simulink model "SMA_Model"  (R2021b)
settings: Solver=VariableStepAuto  StartTime=0.0  StopTime=50.0  FixedStep=1e-6  RelTol=1e-3
values from neighbouring files (symbols this model uses):
  c_heat = 837.36    [Model_Parameters.m]
  do = 5e-4    (= 0.0005)    [Model_Parameters.m]
  h = 70    [Model_Parameters.m]
  i = 0.8    [Model_Parameters.m]
  Initial_Rm = 1    [Model_Parameters.m]
  Initial_temperature = 100    [Model_Parameters.m]
  Lo = 0.98    [Model_Parameters.m]
  mu_minus = 57    [Model_Parameters.m]
  mu_plus = 72    [Model_Parameters.m]
  ni_minus = 1    [Model_Parameters.m]
  ni_plus = 1    [Model_Parameters.m]
  R = 4.3    [Model_Parameters.m]
  rho = 6450    [Model_Parameters.m]
  sigma_minus = 6    [Model_Parameters.m]
  sigma_plus = 6    [Model_Parameters.m]
  Slider_Friction = 0.11    [Model_Parameters.m]
  T_amb = 20    [Model_Parameters.m]
  v = 24    [Model_Parameters.m]
libraries: fl_lib x7, nesl_utility x3
settings Model: Creator=barag  LastModifiedBy=barag

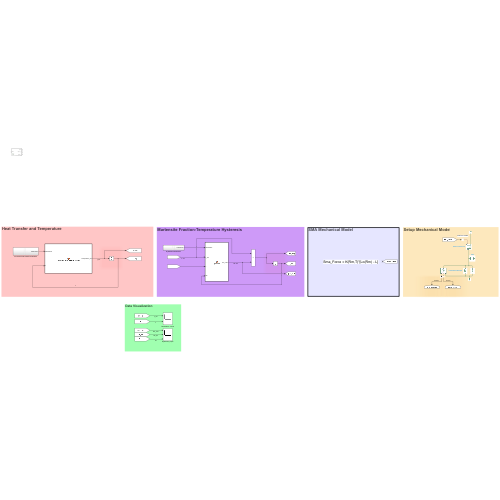
[thumbnail: Simulink's stored preview of the top-level diagram]
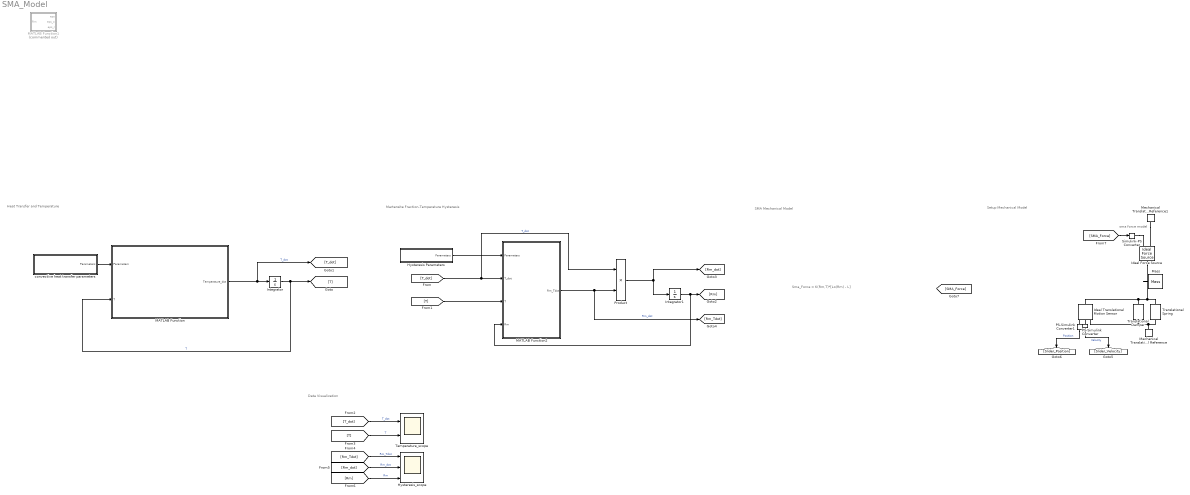
== system SMA_Model ==
  note: Sma_Force = K(Rm,T)*[Lo(Rm) - L]
  note: SMA Mechanical Model
  note: Setup Mechanical Model
  note: sma force model
  note: Data Visualization
  note: Martensite Fraction-Temperature Hysteresis
  note: Heat Transfer and Temperature
  Hysteresis Parameters : Subsystem
  Hysteresis_scope : Scope  NumInputPorts=3
  Ideal Force Source : fl_lib/Mechanical/Mechanical Sources/Ideal Force Source
  Ideal Translational Motion Sensor : fl_lib/Mechanical/Mechanical Sensors/Ideal Translational Motion Sensor  offset=0 m
  Integrator : Integrator  InitialCondition=Initial_temperature
  Integrator1 : Integrator  InitialCondition=Initial_Rm
  MATLAB Function : MATLAB Function  TreatAsAtomicUnit=on
  MATLAB Function1 : MATLAB Function  Commented=on  TreatAsAtomicUnit=on
  MATLAB Function2 : MATLAB Function  TreatAsAtomicUnit=on
  Mass : fl_lib/Mechanical/Translational Elements/Mass  mass=Slider_Mass kg  num_ports=foundation.enum.numPorts2.one  v_specify=off  v_priority=High  v=0 m/s  v_nominal_specify=off  v_nominal_unit=m/s  v_nominal_value=1  f_specify=off  f_priority=None  f=0 N  f_nominal_specify=off  f_nominal_unit=N  f_nominal_value=1
  Mechanical Translational Reference : fl_lib/Mechanical/Translational Elements/Mechanical Translational Reference
  Mechanical Translational Reference1 : fl_lib/Mechanical/Translational Elements/Mechanical Translational Reference
  PS-Simulink Converter : nesl_utility/PS-Simulink Converter  PhysicalDomain=network_engine_domain  SubClassName=ps_output  LeftPortType=input  RightPortType=output  PseudoPeriodic=off  Frequencies=[]  Unit=inherit  AffineConversion=off
      settings: SourceProductBaseCode=PW,SS
  PS-Simulink Converter1 : nesl_utility/PS-Simulink Converter  PhysicalDomain=network_engine_domain  SubClassName=ps_output  LeftPortType=input  RightPortType=output  PseudoPeriodic=off  Frequencies=[]  Unit=inherit  AffineConversion=off
      settings: SourceProductBaseCode=PW,SS
  Product : Product
  Simulink-PS Converter : nesl_utility/Simulink-PS Converter  PhysicalDomain=network_engine_domain  SubClassName=ps_input  LeftPortType=input  RightPortType=output  PseudoPeriodic=off  Frequencies=[]  NoiseDistribution=none  NoiseParameters=[]  Unit=1  AffineConversion=off  FilteringAndDerivatives=provide  SimscapeFilterOrder=1  InputFilterTimeConstant=0.001  UdotUserProvided=0
      settings: SourceProductBaseCode=PW,SS
  Temperature_scope : Scope  NumInputPorts=2
  Translational Damper : fl_lib/Mechanical/Translational Elements/Translational Damper  D=Slider_Friction N/(m/s)  v_specify=off  v_priority=None  v=0 m/s  v_nominal_specify=off  v_nominal_unit=m/s  v_nominal_value=1  f_specify=off  f_priority=None  f=0 N  f_nominal_specify=off  f_nominal_unit=N  f_nominal_value=1
  Translational Spring : fl_lib/Mechanical/Translational Elements/Translational Spring  spr_rate=Spring_Stiff N/m  v_specify=off  v_priority=None  v=0 m/s  v_nominal_specify=off  v_nominal_unit=m/s  v_nominal_value=1  f_specify=off  f_priority=High  f=9 N  f_nominal_specify=off  f_nominal_unit=N  f_nominal_value=1  x_specify=off  x_priority=High  x=0 m  x_nominal_specify=off  x_nominal_unit=m  x_nominal_value=1
  convective heat transfer parameters : Subsystem
  wires:
  MATLAB Function/1(Temperature_dot) -> [T_dot], Integrator/1  "T_dot"
  Integrator/1 -> [T], MATLAB Function/2(T)  "T"
  convective heat transfer parameters/1(Parameters) -> MATLAB Function/1(Parameters)
  Hysteresis Parameters/1(Parameters) -> MATLAB Function2/1(Parameters)
  [T_dot] -> Product/1, MATLAB Function2/2(T_dot)  "T_dot"
  MATLAB Function2/1(Rm_Tdot) -> [Rm_Tdot], Product/2  "Rm_dot"
  [T_dot] -> Temperature_scope/1  "T_dot"
  [T] -> Temperature_scope/2  "T"
  [Rm_Tdot] -> Hysteresis_scope/1  "Rm_Tdot"
  [Rm_dot] -> Hysteresis_scope/2  "Rm_dot"
  [Rm] -> Hysteresis_scope/3  "Rm"
  Integrator1/1 -> [Rm], MATLAB Function2/4(Rm)
  [T] -> MATLAB Function2/3(T)
  Product/1 -> [Rm_dot], Integrator1/1
  PS-Simulink Converter/1 -> [Slider_Velocity]  "Velocity"
  PS-Simulink Converter1/1 -> [Slider_Position]  "Position"
  [SMA_Force] -> Simulink-PS Converter/1
  connections:
  Translational Damper/RConn1 -- Ideal Translational Motion Sensor/RConn1 -- Translational Spring/RConn1 -- Mechanical Translational Reference/LConn1
  Translational Damper/LConn1 -- Ideal Translational Motion Sensor/LConn1 -- Mass/LConn1 -- Ideal Force Source/LConn1 -- Translational Spring/LConn1
  Mechanical Translational Reference1/LConn1 -- Ideal Force Source/RConn2
  PS-Simulink Converter/LConn1 -- Ideal Translational Motion Sensor/RConn2
  PS-Simulink Converter1/LConn1 -- Ideal Translational Motion Sensor/RConn3
  Simulink-PS Converter/RConn1 -- Ideal Force Source/RConn1

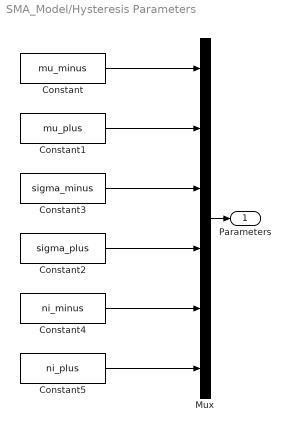
== system SMA_Model/Hysteresis Parameters ==
  Constant : Constant  Value=mu_minus
  Constant1 : Constant  Value=mu_plus
  Constant2 : Constant  Value=sigma_plus
  Constant3 : Constant  Value=sigma_minus
  Constant4 : Constant  Value=ni_minus
  Constant5 : Constant  Value=ni_plus
  Mux : Mux  Inputs=6
  Parameters : Outport
  wires:
  Mux/1 -> Parameters/1
  Constant2/1 -> Mux/4
  Constant/1 -> Mux/1
  Constant4/1 -> Mux/5
  Constant1/1 -> Mux/2
  Constant5/1 -> Mux/6
  Constant3/1 -> Mux/3

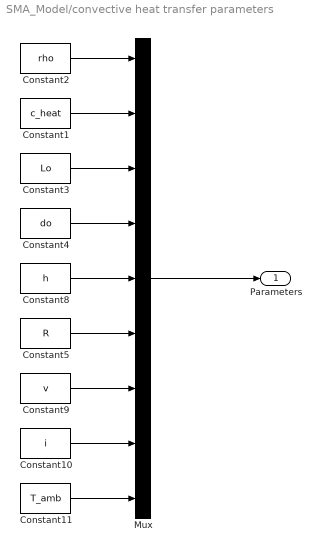
== system SMA_Model/convective heat transfer parameters ==
  Constant1 : Constant  Value=c_heat
  Constant10 : Constant  Value=i
  Constant11 : Constant  Value=T_amb
  Constant2 : Constant  Value=rho
  Constant3 : Constant  Value=Lo
  Constant4 : Constant  Value=do
  Constant5 : Constant  Value=R
  Constant8 : Constant  Value=h
  Constant9 : Constant  Value=v
  Mux : Mux  Inputs=9
  Parameters : Outport
  wires:
  Constant8/1 -> Mux/5
  Constant2/1 -> Mux/1
  Constant1/1 -> Mux/2
  Constant9/1 -> Mux/7
  Constant3/1 -> Mux/3
  Constant11/1 -> Mux/9
  Constant10/1 -> Mux/8
  Constant4/1 -> Mux/4
  Mux/1 -> Parameters/1
  Constant5/1 -> Mux/6

== matlab function SMA_Model/MATLAB Function1 ==
  data: Rm input; eps output; eps_o output; eps_r output
function [eps,eps_o,eps_r]= Epsilon(Rm)

c1 = pi*(do^2)*(Ea + (Em - Ea)*Rm);
d1 = -4*k*Lo - c1*(1-(2*eps_o));
e1 = 4*k*Delta - c1*eps_o*(1-eps_o);

c2 = pi*(do^2)*(Ea + (ET - Ea)*Rm);
d2 = -4*k*Lo -c2*(1-(2*eps_o)) +  pi*(do^2)*Rm*eps_ym*(Em - ET);
e2 = 4*k*Delta -c2*eps_o*(1-eps_o) + Rm*eps_ym*(Em - ET);

c3 = pi*(do^2)*(Ea + (Ed - Ea)*Rm);
d3 = -4*k*Lo -c3*(1-(2*eps_o)) + pi*(do^2)*Rm*(eps_ym*(Em - ET) + eps_dm*(ET - Ed));
e3 = 4*k*Delta -c3*eps_o*(1-eps_o) + Rm*(eps_ym*(Em - ET) + eps_dm*(ET - Ed));



Epsilon = 0;

== matlab function SMA_Model/MATLAB Function ==
  data: Parameters input; Temperature_dot output; T input
function Temperature_dot = Convective_Heat_Transfer_Equation(Parameters, T)
% Parameters Estraztion
rho =    Parameters(1); % mass density of SMA wire[kgm-3]
c_heat = Parameters(2); % specific heat of SMA wire [Jkg-1C-1]
Lo =     Parameters(3); % undeformed SMA wire length in 100% state [m]
do =     Parameters(4); % cross-sectional diameter of undeformed SMA wire [m]
h =      Parameters(5); % convection heat transfer coefficient [Wm-2C-1]
R =      Parameters(6)*Lo; % SMA electric resistance per unit lenght [Ohm/m] * Lo
v =      Parameters(7); % voltage across SMA wire [V]
i =      Parameters(8); % current through SMA wire [A]
T_amb =  Parameters(9); % ambient temperature [C]

% Equation Terms Definitions:
Term_1 = (rho*c_heat*pi*Lo*(do^2))/4;
%Term_2 = (1+(eps/2))*p1*do*Lo*h;
Term_2_simplified = pi*do*Lo*h;
El_Pow_Term = R*(i^2);
T_diff = T - T_amb;

% Temperature Rate of Variation :
Temperature_dot = (El_Pow_Term - Term_2_simplified*T_diff)/Term_1; %
%Simplified version with eps assumed to be small and neglectable
%Temperature_dot = (El_Pow_Term - Term_2*T_diff)/Term_1;

== matlab function SMA_Model/MATLAB Function2 ==
  data: Parameters input; Rm_Tdot output; T_dot input; T input; Rm input
function Rm_Tdot = Hysteresis(Parameters, T_dot, T, Rm)
    % Parameter Extraction
    mu_minus =    Parameters(1);
    mu_plus =     Parameters(2);
    sigma_minus = Parameters(3);
    sigma_plus =  Parameters(4);
    ni_minus =    Parameters(5);
    ni_plus =     Parameters(6);

    ER_minus = erf((T-mu_minus)/(sigma_minus*sqrt(2)));
    ER_plus = erf((T-mu_plus)/(sigma_plus*sqrt(2)));

    H_minus = 0.5 * (1 + ER_minus);
    H_plus  = 0.5 * (1 + ER_plus);

    Exp_minus = exp(-((T-mu_minus)/(sigma_minus*sqrt(2)))^2);
    Exp_plus  = exp(-((T-mu_plus)/(sigma_plus*sqrt(2)))^2);

    Gauss_minus= (1/(sigma_minus*sqrt(2*pi)))*Exp_minus;
    Gauss_plus = (1/(sigma_plus*sqrt(2*pi)))*Exp_plus;
    
    Rm_Tdot=0;
    if T_dot >= 0
        ceff_plus = (H_minus + Rm - 1)/(H_plus - H_minus);
        Rm_Tdot = ceff_plus*Gauss_plus*ni_plus;  
    elseif T_dot < 0
        ceff_minus = (H_plus + Rm - 1)/(H_minus - H_plus);
        Rm_Tdot = ceff_minus*Gauss_minus*ni_minus;
    end 
%   if Rm_Tdot == 0
%       Rm_Tdot = 1e-6;
%   end
end
